simulink model "VehicleSteering_sim"  (R2018b)
settings: Solver=VariableStepAuto  StartTime=0.0  StopTime=10.0  RelTol=1e-3
values from neighbouring files (symbols this model uses):
  A = Ag    [Example_VehicleSteering_Integral_action.m]
  B = Bg    [Example_VehicleSteering_Integral_action.m]
  C = eye(3)    [Example_VehicleSteering_Integral_action.m]
  D = [0 0 0]'    [Example_VehicleSteering_Integral_action.m]
  K = [p - ap] * Wr_tilde * Wr^(-1)    [Example_VehicleSteering_Integral_action.m]
  kr = 1    [Example_VehicleSteering_Integral_action.m]
settings Model: Creator=jofr  LastModifiedBy=rodralez
settings DebuggingCC: ArithmeticOperatorsInVariantConditions=warning
settings SFSimCC: SimUseLocalCustomCode=off  CustomCodeUndefinedFunction=UseInterfaceOnly
settings RTWCC: RTWUseLocalCustomCode=off

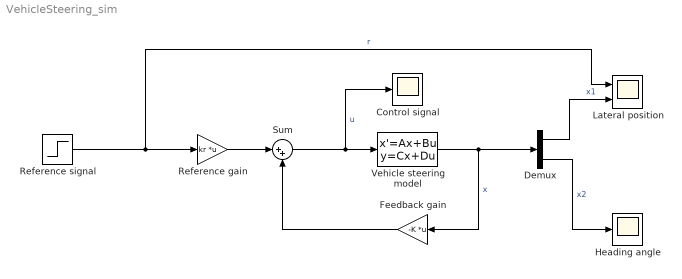
== system VehicleSteering_sim ==
  Control signal : Scope
  Demux : Demux  Outputs=2
  Feedback gain : Gain  Gain=-K  Multiplication=Matrix(K*u)
  Heading angle : Scope
  Lateral position : Scope  NumInputPorts=2
  Reference gain : Gain  Gain=kr  Multiplication=Matrix(K*u)
  "Reference signal " : Step  SampleTime=0
  Sum : Sum  Inputs=|++
  Vehicle steering model : StateSpace  A=A  B=B  C=C  D=D  InitialCondition=0
  wires:
  Vehicle steering model/1 -> Demux/1, Feedback gain/1  "x"
  Sum/1 -> Control signal/1, Vehicle steering model/1  "u"
  Feedback gain/1 -> Sum/2
  Reference gain/1 -> Sum/1
  Demux/2 -> Heading angle/1  "x2"
  "Reference signal "/1 -> Lateral position/1, Reference gain/1  "r"
  Demux/1 -> Lateral position/2  "x1"
